simulink model "planPath_sim"  (R2020a)
settings: Solver=FixedStepDiscrete  StartTime=0.0  StopTime=100  FixedStep=TS  RelTol=1e-3  EnableMultiTasking=on
PostLoadFcn:
  | params
model workspace (MAT data in the model file):
  Ia = 0.1
  Id = 0.25
  Pa = 5
  Pd = 9
  TS = 0.01
undefined symbols (not defined in the file): DiscIntNeverNeededParam, L, r, StartTheta, StartX, StartY
libraries: simulink_extras x3, simulink x2
settings Model: EnablePacing=on  Creator=mgovinda  LastModifiedBy=mmarathe
settings DataIOCC: LimitDataPoints=on  SaveFormat=Array  ReturnWorkspaceOutputs=off
settings OptimizationCC: LifeSpan=inf
settings DebuggingCC: UnderspecifiedInitializationDetection=Classic  MergeDetectMultiDrivingBlocksExec=none  SFUnexpectedBacktrackingDiag=warning  SFNoUnconditionalDefaultTransitionDiag=warning  SFExecutionAtInitializationDiag=none  ArithmeticOperatorsInVariantConditions=warning
settings HardwareCC: ProdBitPerPointer=32  ProdBitPerSizeT=32  ProdBitPerPtrDiffT=32  ProdLargestAtomicFloat=None  ProdIntDivRoundTo=Undefined  ProdEndianess=Unspecified  ProdWordSize=32  ProdHWDeviceType=32-bit Generic
settings ModelReferenceCC: PropagateSignalLabelsOutOfModel=off
settings SFSimCC: SimUseLocalCustomCode=off  CustomCodeUndefinedFunction=UseInterfaceOnly
settings RTWCC: RTWUseLocalCustomCode=off
settings CodeAppCC: StateflowObjectComments=on
settings GRTTargetCC: TargetLangStandard=C89/C90 (ANSI)
settings ConfigComp: CovMetricSettings=dw  CovHtmlReporting=on  CovSaveCumulativeToWorkspaceVar=on  CovSaveSingleToWorkspaceVar=on  CovExternalEMLEnable=off

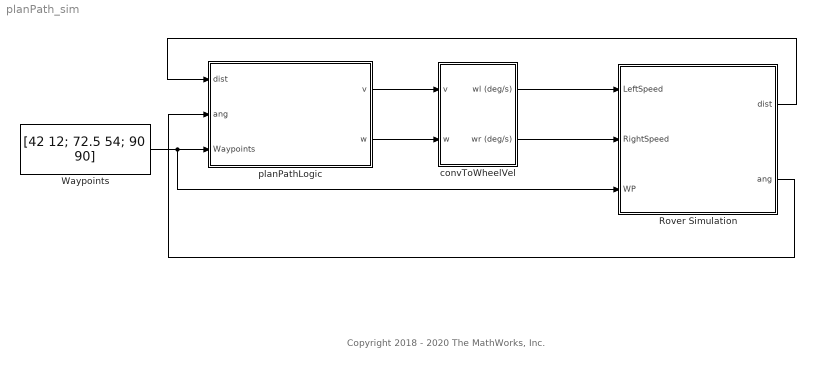
== system planPath_sim ==
  note: Copyright 2018 - 2020 The MathWorks, Inc.
  Rover Simulation : Subsystem
  Waypoints : Constant  Value=[42 12; 72.5 54; 90 90]
  convToWheelVel : Subsystem
  planPathLogic : Stateflow chart  TreatAsAtomicUnit=on
  wires:
  planPathLogic/1(v) -> convToWheelVel/1(v)
  planPathLogic/2(w) -> convToWheelVel/2(w)
  Rover Simulation/1(dist) -> planPathLogic/1(dist)
  Rover Simulation/2(ang) -> planPathLogic/2(ang)
  convToWheelVel/1(wl (deg/s)) -> Rover Simulation/1(LeftSpeed)
  convToWheelVel/2(wr (deg/s)) -> Rover Simulation/2(RightSpeed)
  Waypoints/1 -> Rover Simulation/3(WP), planPathLogic/3(Waypoints)

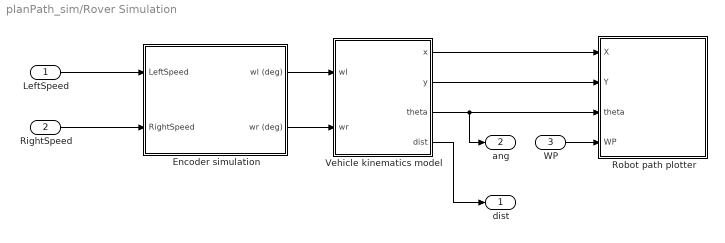
== system planPath_sim/Rover Simulation ==
  LeftSpeed : Inport
  RightSpeed : Inport  Port=2
  WP : Inport  Port=3
  " Encoder simulation" : Subsystem
  Robot path plotter : Subsystem
  "Vehicle kinematics model " : Subsystem
  dist : Outport  VectorParamsAs1DForOutWhenUnconnected=off
  ang : Outport  Port=2  VectorParamsAs1DForOutWhenUnconnected=off
  wires:
  "Vehicle kinematics model "/1(x) -> Robot path plotter/1(X)
  "Vehicle kinematics model "/2(y) -> Robot path plotter/2(Y)
  "Vehicle kinematics model "/3(theta) -> ang/1, Robot path plotter/3(theta)
  LeftSpeed/1 -> " Encoder simulation"/1(LeftSpeed)
  RightSpeed/1 -> " Encoder simulation"/2(RightSpeed)
  " Encoder simulation"/1(wl (deg)) -> "Vehicle kinematics model "/1(wl)
  " Encoder simulation"/2(wr (deg)) -> "Vehicle kinematics model "/2(wr)
  "Vehicle kinematics model "/4(dist) -> dist/1
  WP/1 -> Robot path plotter/4(WP)

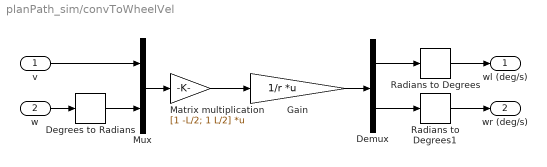
== system planPath_sim/convToWheelVel ==
  v : Inport
  w : Inport  Port=2
  " Gain" : Gain  Gain=1/r  Multiplication=Matrix(K*u)
  Degrees to Radians : simulink_extras/Transformations/Degrees to Radians
  Demux : Demux  Outputs=2
  Matrix multiplication : Gain  Gain=[1 -L/2; 1 L/2]  Multiplication=Matrix(K*u)
  Mux : Mux  Inputs=2
  Radians to Degrees : simulink_extras/Transformations/Radians to Degrees
  Radians to Degrees1 : simulink_extras/Transformations/Radians to Degrees
  wl (deg/s) : Outport  VectorParamsAs1DForOutWhenUnconnected=off
  wr (deg/s) : Outport  Port=2  VectorParamsAs1DForOutWhenUnconnected=off
  wires:
  " Gain"/1 -> Demux/1
  Matrix multiplication/1 -> " Gain"/1
  v/1 -> Mux/1
  Mux/1 -> Matrix multiplication/1
  Demux/1 -> Radians to Degrees/1
  Demux/2 -> Radians to Degrees1/1
  w/1 -> Degrees to Radians/1
  Radians to Degrees/1 -> wl (deg/s)/1
  Radians to Degrees1/1 -> wr (deg/s)/1
  Degrees to Radians/1 -> Mux/2

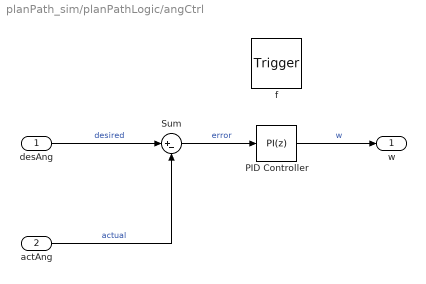
== system planPath_sim/planPathLogic/angCtrl ==
  desAng : Inport  OutDataTypeStr=double  PortDimensions=1
  actAng : Inport  Port=2  OutDataTypeStr=double  PortDimensions=1
  f : TriggerPort  TriggerType=function-call  VariantControl=(inherit)
      settings: CopyFcn=Stateflow.SLINSF.SimulinkMan.removeBlockPreDeleteFcn  PreDeleteFcn=Stateflow.SLINSF.SimulinkMan.unsafePredeleteFcn
  PID Controller : simulink/Continuous/PID Controller  Controller=PI  Form=Parallel  TimeDomain=Discrete-time  UseExternalTs=off  SampleTime=-1  IntegratorMethod=Forward Euler  FilterMethod=Forward Euler  ControllerParametersSource=internal  P=1.25  I=0.25  D=0  UseFilter=on  N=100  TunerSelectOption=Transfer Function Based (PID Tuner App)  InitialConditionSource=internal  InitialConditionForIntegrator=0  InitialConditionForFilter=0  DifferentiatorICPrevScaledInput=0  ExternalReset=none  TrackingMode=off  Kt=1  LimitOutput=off  UpperSaturationLimit=inf  LowerSaturationLimit=-inf  LinearizeAsGain=on  AntiWindupMode=none  Kb=1  POutMin=[]  POutMax=[]  IOutMin=[]  IOutMax=[]  DOutMin=[]  DOutMax=[]  NOutMin=[]  NOutMax=[]  SumOutMin=[]  SumOutMax=[]  SaturationOutMin=[]  SaturationOutMax=[]  PParamMin=[]  PParamMax=[]  IParamMin=[]  IParamMax=[]  DParamMin=[]  DParamMax=[]  NParamMin=[]  NParamMax=[]  KbParamMin=[]  KbParamMax=[]  KtParamMin=[]  KtParamMax=[]  KbOutMin=[]  KbOutMax=[]  KtOutMin=[]  KtOutMax=[]  IntegratorOutMin=[]  IntegratorOutMax=[]  FilterOutMin=[]  FilterOutMax=[]  SumI1OutMin=[]  SumI1OutMax=[]  SumI2OutMin=[]  SumI2OutMax=[]  SumI3OutMin=[]  SumI3OutMax=[]  SumI4OutMin=[]  SumI4OutMax=[]  SumDOutMin=[]  SumDOutMax=[]  DifferentiatorOutMin=[]  DifferentiatorOutMax=[]  FilterDiffOutCoefMin=[]  FilterDiffOutCoefMax=[]  ReciprocalOutMin=[]  ReciprocalOutMax=[]  SumDenOutMin=[]  SumDenOutMax=[]  SumNumOutMin=[]  SumNumOutMax=[]  DivideOutMin=[]  DivideOutMax=[]  UdiffTsProdOutMin=[]  UdiffTsProdOutMax=[]  NTsProdOutMin=[]  NTsProdOutMax=[]  UintegralTsProdOutMin=[]  UintegralTsProdOutMax=[]  UngainTsProdOutMin=[]  UngainTsProdOutMax=[]  IntegratorContinuousStateAttributes=''  IntegratorStateMustResolveToSignalObject=off  IntegratorRTWStateStorageClass=Auto  FilterContinuousStateAttributes=''  FilterStateMustResolveToSignalObject=off  FilterRTWStateStorageClass=Auto  ParallelPVariant=InternalParameters  IdealPVariant=Disabled  IVariant=InternalParameters  DVariant=Disabled  IntegratorVariant=Discrete  SatVariant=Disabled  AWVariant=Passthrough  PCopyVariant=Disabled  TRVariant=Disabled  FdbkBlocksVariant=Forward  IdealPFdbkVariant=Disabled  SatFdbkVariant=Disabled  DerivativeFilterVariant=Disabled  NVariant=Disabled  NCopyVariant=Disabled_SignalSpec  FilterICVariant=Disabled  IntegratorICVariant=InternalICs  ExternalResetVariant=Disabled  TRSumVariant=Passthrough  SumFdbkVariant=Disabled  SumVariant=Sum_PI  TsampFilterVariant=InternalTs  TsampNgainVariant=Passthrough  TsampIntegralVariant=Passthrough
  Sum : Sum  Inputs=|+-
  w : Outport  VectorParamsAs1DForOutWhenUnconnected=off
  wires:
  actAng/1 -> Sum/2  "actual"
  desAng/1 -> Sum/1  "desired"
  PID Controller/1 -> w/1  "w"
  Sum/1 -> PID Controller/1  "error"

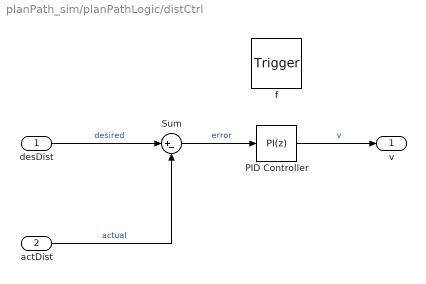
== system planPath_sim/planPathLogic/distCtrl ==
  desDist : Inport  OutDataTypeStr=double  PortDimensions=1
  actDist : Inport  Port=2  OutDataTypeStr=double  PortDimensions=1
  f : TriggerPort  TriggerType=function-call  VariantControl=(inherit)
      settings: CopyFcn=Stateflow.SLINSF.SimulinkMan.removeBlockPreDeleteFcn  PreDeleteFcn=Stateflow.SLINSF.SimulinkMan.unsafePredeleteFcn
  PID Controller : simulink/Continuous/PID Controller  Controller=PI  Form=Parallel  TimeDomain=Discrete-time  UseExternalTs=off  SampleTime=-1  IntegratorMethod=Forward Euler  FilterMethod=Forward Euler  ControllerParametersSource=internal  P=0.25  I=0.05  D=0  UseFilter=on  N=100  TunerSelectOption=Transfer Function Based (PID Tuner App)  InitialConditionSource=internal  InitialConditionForIntegrator=0  InitialConditionForFilter=0  DifferentiatorICPrevScaledInput=0  ExternalReset=none  TrackingMode=off  Kt=1  LimitOutput=off  UpperSaturationLimit=inf  LowerSaturationLimit=-inf  LinearizeAsGain=on  AntiWindupMode=none  Kb=1  POutMin=[]  POutMax=[]  IOutMin=[]  IOutMax=[]  DOutMin=[]  DOutMax=[]  NOutMin=[]  NOutMax=[]  SumOutMin=[]  SumOutMax=[]  SaturationOutMin=[]  SaturationOutMax=[]  PParamMin=[]  PParamMax=[]  IParamMin=[]  IParamMax=[]  DParamMin=[]  DParamMax=[]  NParamMin=[]  NParamMax=[]  KbParamMin=[]  KbParamMax=[]  KtParamMin=[]  KtParamMax=[]  KbOutMin=[]  KbOutMax=[]  KtOutMin=[]  KtOutMax=[]  IntegratorOutMin=[]  IntegratorOutMax=[]  FilterOutMin=[]  FilterOutMax=[]  SumI1OutMin=[]  SumI1OutMax=[]  SumI2OutMin=[]  SumI2OutMax=[]  SumI3OutMin=[]  SumI3OutMax=[]  SumI4OutMin=[]  SumI4OutMax=[]  SumDOutMin=[]  SumDOutMax=[]  DifferentiatorOutMin=[]  DifferentiatorOutMax=[]  FilterDiffOutCoefMin=[]  FilterDiffOutCoefMax=[]  ReciprocalOutMin=[]  ReciprocalOutMax=[]  SumDenOutMin=[]  SumDenOutMax=[]  SumNumOutMin=[]  SumNumOutMax=[]  DivideOutMin=[]  DivideOutMax=[]  UdiffTsProdOutMin=[]  UdiffTsProdOutMax=[]  NTsProdOutMin=[]  NTsProdOutMax=[]  UintegralTsProdOutMin=[]  UintegralTsProdOutMax=[]  UngainTsProdOutMin=[]  UngainTsProdOutMax=[]  IntegratorContinuousStateAttributes=''  IntegratorStateMustResolveToSignalObject=off  IntegratorRTWStateStorageClass=Auto  FilterContinuousStateAttributes=''  FilterStateMustResolveToSignalObject=off  FilterRTWStateStorageClass=Auto  ParallelPVariant=InternalParameters  IdealPVariant=Disabled  IVariant=InternalParameters  DVariant=Disabled  IntegratorVariant=Discrete  SatVariant=Disabled  AWVariant=Passthrough  PCopyVariant=Disabled  TRVariant=Disabled  FdbkBlocksVariant=Forward  IdealPFdbkVariant=Disabled  SatFdbkVariant=Disabled  DerivativeFilterVariant=Disabled  NVariant=Disabled  NCopyVariant=Disabled_SignalSpec  FilterICVariant=Disabled  IntegratorICVariant=InternalICs  ExternalResetVariant=Disabled  TRSumVariant=Passthrough  SumFdbkVariant=Disabled  SumVariant=Sum_PI  TsampFilterVariant=InternalTs  TsampNgainVariant=Passthrough  TsampIntegralVariant=Passthrough
  Sum : Sum  Inputs=|+-
  v : Outport  VectorParamsAs1DForOutWhenUnconnected=off
  wires:
  actDist/1 -> Sum/2  "actual"
  desDist/1 -> Sum/1  "desired"
  PID Controller/1 -> v/1  "v"
  Sum/1 -> PID Controller/1  "error"

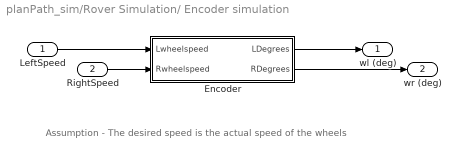
== system planPath_sim/Rover Simulation/ Encoder simulation ==
  note: Assumption - The desired speed is the actual speed of the wheels
  LeftSpeed : Inport
  RightSpeed : Inport  Port=2
  Encoder : Subsystem
  wl (deg) : Outport  VectorParamsAs1DForOutWhenUnconnected=off
  wr (deg) : Outport  Port=2  VectorParamsAs1DForOutWhenUnconnected=off
  wires:
  Encoder/1(LDegrees) -> wl (deg)/1
  Encoder/2(RDegrees) -> wr (deg)/1
  RightSpeed/1 -> Encoder/2(Rwheelspeed)
  LeftSpeed/1 -> Encoder/1(Lwheelspeed)

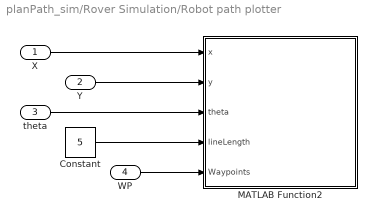
== system planPath_sim/Rover Simulation/Robot path plotter ==
  X : Inport
  Y : Inport  Port=2
  theta : Inport  Port=3
  WP : Inport  Port=4
  Constant : Constant  Value=5
  MATLAB Function2 : MATLAB Function  TreatAsAtomicUnit=on
  wires:
  Constant/1 -> MATLAB Function2/4(lineLength)
  X/1 -> MATLAB Function2/1(x)
  Y/1 -> MATLAB Function2/2(y)
  theta/1 -> MATLAB Function2/3(theta)
  WP/1 -> MATLAB Function2/5(Waypoints)

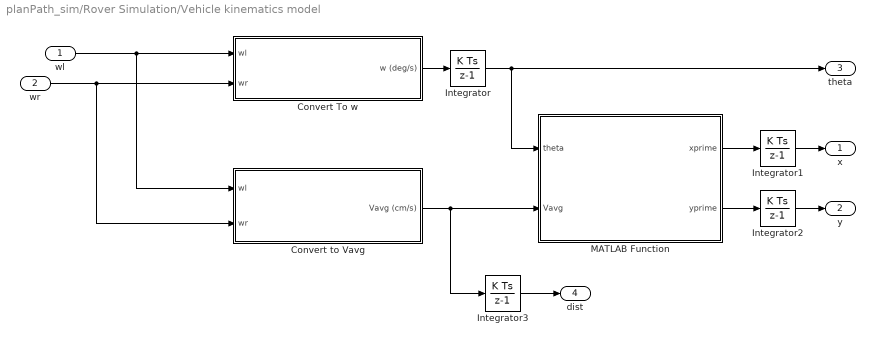
== system planPath_sim/Rover Simulation/Vehicle kinematics model  ==
  wl : Inport
  wr : Inport  Port=2
  Convert To w : Subsystem
  Convert to Vavg : Subsystem
  Integrator : DiscreteIntegrator  gainval=1  InitialCondition=StartTheta  SampleTime=-1  ICPrevOutput=DiscIntNeverNeededParam  ICPrevScaledInput=DiscIntNeverNeededParam
  Integrator1 : DiscreteIntegrator  gainval=1  InitialCondition=StartX  SampleTime=-1  ICPrevOutput=DiscIntNeverNeededParam  ICPrevScaledInput=DiscIntNeverNeededParam
  Integrator2 : DiscreteIntegrator  gainval=1  InitialCondition=StartY  SampleTime=-1  ICPrevOutput=DiscIntNeverNeededParam  ICPrevScaledInput=DiscIntNeverNeededParam
  Integrator3 : DiscreteIntegrator  gainval=1  SampleTime=-1  ICPrevOutput=DiscIntNeverNeededParam  ICPrevScaledInput=DiscIntNeverNeededParam
  MATLAB Function : MATLAB Function  TreatAsAtomicUnit=on
  x : Outport  VectorParamsAs1DForOutWhenUnconnected=off
  y : Outport  Port=2  VectorParamsAs1DForOutWhenUnconnected=off
  theta : Outport  Port=3  VectorParamsAs1DForOutWhenUnconnected=off
  dist : Outport  Port=4  VectorParamsAs1DForOutWhenUnconnected=off
  wires:
  MATLAB Function/1(xprime) -> Integrator1/1
  MATLAB Function/2(yprime) -> Integrator2/1
  Integrator1/1 -> x/1
  Integrator2/1 -> y/1
  Integrator/1 -> theta/1, MATLAB Function/1(theta)
  wl/1 -> Convert to Vavg/1(wl), Convert To w/1(wl)
  wr/1 -> Convert to Vavg/2(wr), Convert To w/2(wr)
  Convert to Vavg/1(Vavg (cm/s)) -> Integrator3/1, MATLAB Function/2(Vavg)
  Convert To w/1(w (deg/s)) -> Integrator/1
  Integrator3/1 -> dist/1

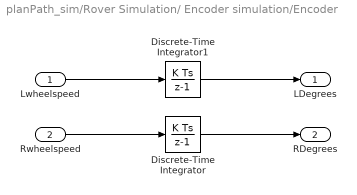
== system planPath_sim/Rover Simulation/ Encoder simulation/Encoder ==
  Lwheelspeed : Inport
  Rwheelspeed : Inport  Port=2
  Discrete-Time Integrator : DiscreteIntegrator  SampleTime=-1  ICPrevOutput=DiscIntNeverNeededParam  ICPrevScaledInput=DiscIntNeverNeededParam
  Discrete-Time Integrator1 : DiscreteIntegrator  SampleTime=-1  ICPrevOutput=DiscIntNeverNeededParam  ICPrevScaledInput=DiscIntNeverNeededParam
  LDegrees : Outport  VectorParamsAs1DForOutWhenUnconnected=off
  RDegrees : Outport  Port=2  VectorParamsAs1DForOutWhenUnconnected=off
  wires:
  Rwheelspeed/1 -> Discrete-Time Integrator/1
  Lwheelspeed/1 -> Discrete-Time Integrator1/1
  Discrete-Time Integrator/1 -> RDegrees/1
  Discrete-Time Integrator1/1 -> LDegrees/1

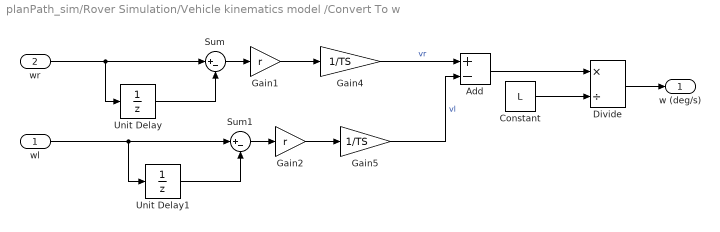
== system planPath_sim/Rover Simulation/Vehicle kinematics model /Convert To w ==
  wl : Inport
  wr : Inport  Port=2
  Add : Sum  Inputs=+-
  Constant : Constant  Value=L
  Divide : Product  Inputs=*/
  Gain1 : Gain  Gain=r
  Gain2 : Gain  Gain=r
  Gain4 : Gain  Gain=1/TS
  Gain5 : Gain  Gain=1/TS
  Sum : Sum  Inputs=|+-
  Sum1 : Sum  Inputs=|+-
  Unit Delay : UnitDelay  SampleTime=-1  HasFrameUpgradeWarning=on
  Unit Delay1 : UnitDelay  SampleTime=-1  HasFrameUpgradeWarning=on
  w (deg/s) : Outport  VectorParamsAs1DForOutWhenUnconnected=off
  wires:
  Unit Delay1/1 -> Sum1/2
  Sum1/1 -> Gain2/1
  wl/1 -> Unit Delay1/1, Sum1/1
  wr/1 -> Sum/1, Unit Delay/1
  Sum/1 -> Gain1/1
  Unit Delay/1 -> Sum/2
  Gain1/1 -> Gain4/1
  Gain2/1 -> Gain5/1
  Add/1 -> Divide/1
  Constant/1 -> Divide/2
  Gain4/1 -> Add/1  "vr"
  Gain5/1 -> Add/2  "vl"
  Divide/1 -> w (deg/s)/1

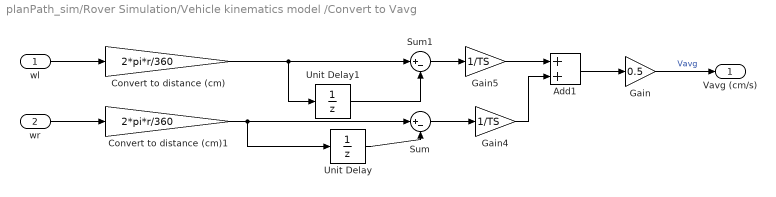
== system planPath_sim/Rover Simulation/Vehicle kinematics model /Convert to Vavg ==
  wl : Inport
  wr : Inport  Port=2
  Add1 : Sum
  Convert to distance (cm) : Gain  Gain=2*pi*r/360
  Convert to distance (cm)1 : Gain  Gain=2*pi*r/360
  Gain : Gain  Gain=0.5
  Gain4 : Gain  Gain=1/TS
  Gain5 : Gain  Gain=1/TS
  Sum : Sum  Inputs=|+-
  Sum1 : Sum  Inputs=|+-
  Unit Delay : UnitDelay  SampleTime=-1  HasFrameUpgradeWarning=on
  Unit Delay1 : UnitDelay  SampleTime=-1  HasFrameUpgradeWarning=on
  Vavg (cm/s) : Outport  VectorParamsAs1DForOutWhenUnconnected=off
  wires:
  Gain/1 -> Vavg (cm/s)/1  "Vavg"
  Add1/1 -> Gain/1
  Unit Delay/1 -> Sum/2
  Sum/1 -> Gain4/1
  wr/1 -> Convert to distance (cm)1/1
  Gain4/1 -> Add1/2
  Gain5/1 -> Add1/1
  Sum1/1 -> Gain5/1
  Unit Delay1/1 -> Sum1/2
  wl/1 -> Convert to distance (cm)/1
  Convert to distance (cm)/1 -> Unit Delay1/1, Sum1/1
  Convert to distance (cm)1/1 -> Unit Delay/1, Sum/1

== matlab function planPath_sim/Rover Simulation/Vehicle kinematics model /MATLAB Function ==
  settings: updateMethod=DISCRETE  sampleTime=TS
  data: xprime output; yprime output; theta input; Vavg input
function [xprime, yprime] = vehiclesPath(theta, Vavg)
%#codegen

xprime = Vavg*cosd(theta);
yprime = Vavg*sind(theta);

== stateflow chart planPath_sim/planPathLogic ==
  state StopFirst
    entry:
    v = 0; w= 0;
  state Turn
    entry:
    desAng = calcAngle(nextWPIndex);
    during, exit:
    v = 0;
    w = angCtrl(desAng,ang);
  state MoveForward
    entry:
    desDist = calcDist(nextWPIndex)+dist;
    during, exit:
    v = distCtrl(desDist, dist);
    w = 0;
  state w = angCtrl(desAng,actAng) [function]
  state v = distCtrl(desDist,actDist) [function]
  state Stop
    entry:
    v = 0;
    w = 0;
  (default) -> StopFirst
  StopFirst -> Turn : after(1,sec)
  Turn -> MoveForward : [abs(desAng - ang) < 0.5]
  MoveForward -> (junction 101) : [abs(desDist - dist) < 0.1]{nextWPIndex = nextWPIndex+1}
  (junction 101) -> Turn [order 2]
  (junction 101) -> Stop [order 1] : [nextWPIndex == size(Waypoints,1)]
  data: desAngle function_output; Index function_input; desDistance function_output; Index function_input; desAng function_input double size=1; actAng function_input double size=1; w function_output; desDist function_input double size=1; actDist function_input double size=1; v function_output; dist input; ang input; v output double size=1; w output double size=1; desDist local; desAng local; Waypoints input; nextWPIndex local =1
  function desAngle  = calcAngle(Index):
    | function desAngle  = calcAngle(Index)
    | 
    | % Determine the distance between the rover and the waypoint
    | toReachX = Waypoints(Index+1,1);
    | toReachY = Waypoints(Index+1,2);
    | x = Waypoints(Index,1);
    | y = Waypoints(Index,2);
    | distX = toReachX - x;
    | distY = toReachY - y;
    | 
    | % Determine which quadrant the target is in
    | if distX > 0 && distY >= 0
    |     quadrant = 1;
    | elseif distX <= 0 && distY > 0
    |     quadrant = 2;
    | elseif distX < 0 && distY <= 0
    |     quadrant = 3;
    | elseif distX >= 0 && distY < 0
    |     quadrant = 4;
    | else
    |     quadrant = 0;
    | end
    | 
    | % Determine the desired heading for the rover
    | desAngle = atand((toReachY-y)/(toReachX-x));
    | 
    | % Add corrections based upon which quadrant the target is in
    | switch quadrant
    |     case 1
    |         
    |     case 2
    |         desAngle = 180 - abs(desAngle);
    |     case 3
    |         desAngle = 180 + desAngle;
    |     case 4
    |         desAngle = 360 + desAngle;
    |     otherwise 
    |         desAngle = 0;
    | end
    | 
    | % Ensure that the angle always remains between 0-360 degrees 
    | if desAngle > 360 
    |     desAngle = desAngle - 360;
    | end
    | end
  function desDistance = calcDist(Index):
    | function desDistance = calcDist(Index)
    | 
    | % Determine the distance between the rover and the waypoint
    | toReachX = Waypoints(Index+1,1);
    | toReachY = Waypoints(Index+1,2);
    | x = Waypoints(Index,1);
    | y = Waypoints(Index,2);
    | distX = toReachX - x;
    | distY = toReachY - y;
    | 
    | % Determine the distance that the rover should travel to reach the waypoint
    | desDistance = sqrt(distX^2+distY^2);
    | end

== matlab function planPath_sim/Rover Simulation/Robot path plotter/MATLAB Function2 ==
  data: x input; y input; theta input; lineLength input; StartX parameter; StartY parameter; StartTheta parameter; Waypoints input
function plotRobotAndWP(x,y,theta,lineLength, StartX, StartY, StartTheta, Waypoints)

persistent h h1 h2;
if isempty(h)
    h = figure('name','Map of the Robot');
    h1 = plot(StartX,StartY,'bo');
    hold on
    xlim([0 100])
    ylim([0 100])
    xp = [StartX StartX+lineLength*cosd(StartTheta)];
    yp = [StartY StartY+lineLength*sind(StartTheta)];
    h2 = plot(xp,yp,'b');
    for i = 2:size(Waypoints,1)-1
        plot(Waypoints(i,1),Waypoints(i,2),'ro')
    end
    plot(Waypoints(end,1),Waypoints(end,2),'go')
    hold off
end

set(h1,'xdata',x,'ydata',y)
xp = [x x+lineLength*cosd(theta)];
yp = [y y+lineLength*sind(theta)];
set(h2,'xdata',xp,'ydata',yp)
drawnow('limitrate')
